simulink model "sampleModel133"  (R2021b)
settings: Solver=VariableStepAuto  StartTime=0.0  StopTime=10.0  RelTol=1e-3
libraries: simulink x4
settings Model: Creator=user  LastModifiedBy=user

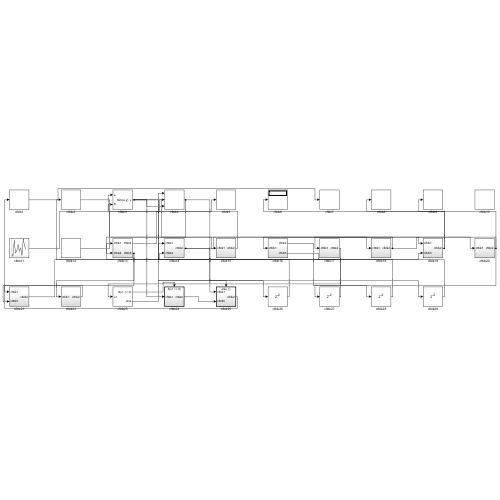
[thumbnail: Simulink's stored preview of the top-level diagram]
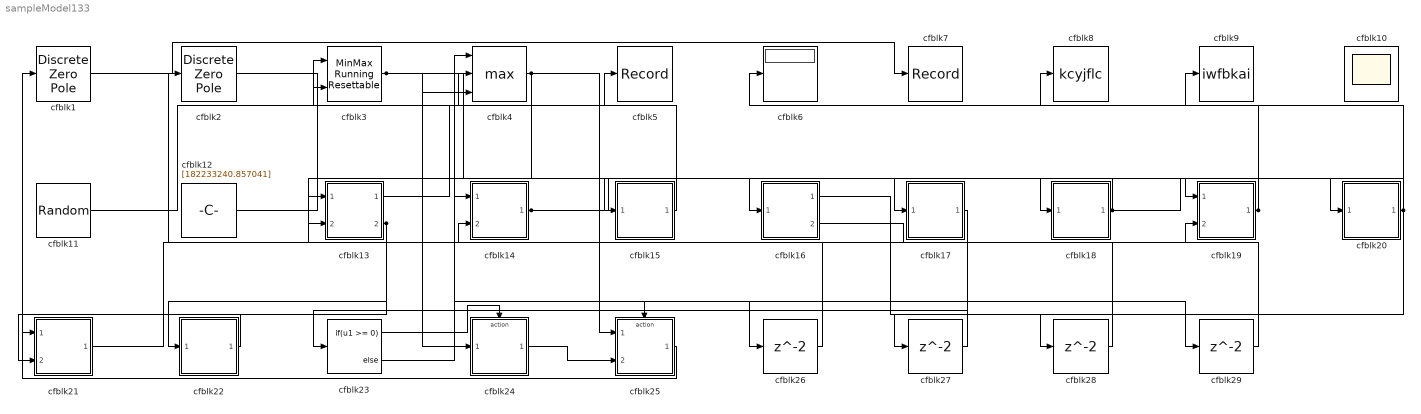
== system sampleModel133 ==
  cfblk1 : DiscreteZeroPole  Poles=[0 0.5]  Gain=1
  cfblk10 : Scope
      settings: Floating=on
  cfblk11 : UniformRandomNumber  Minimum=[-6625192953.180672]  Maximum=[659722112.246496]  Seed=[92829086.000000]  SampleTime=0.1
  cfblk12 : Constant  Value=[182233240.857041]  SampleTime=1
  cfblk13 : Subsystem
  cfblk14 : Subsystem
  cfblk15 : Subsystem
  cfblk16 : Subsystem
  cfblk17 : Subsystem
  cfblk18 : Subsystem
  cfblk19 : Subsystem
  cfblk2 : DiscreteZeroPole  Poles=[0 0.5]  Gain=1
  cfblk20 : Subsystem
  cfblk21 : Subsystem
  cfblk22 : Subsystem
  cfblk23 : If  IfExpression=u1 >= 0  SampleTime=1
  cfblk24 : Subsystem  TreatAsAtomicUnit=on
  cfblk25 : Subsystem  TreatAsAtomicUnit=on
  cfblk{26..29} (4 alike) : Delay  SampleTime=1
  cfblk3 : simulink/Math Operations/MinMax Running Resettable  Function=min  vinit=0.0
  cfblk4 : MinMax  Function=max  Inputs=3
  cfblk5 : Record  FileSettingsInternal="{\"entries\":[{\"content\":{\"excelSettings\":{\"content\":{},\"type\":\"Streamout.ExcelSettings\"}},\"type\":\"Streamout.FileSettingStorage\",\"uuid\":\"0f116b82-28e0-41c1-9d28-ccf6914d8969\"}],\"packageUris\":[\"http://schema.mathworks.com/mf0/streamout_blocks/R2020a\"],\"version\":\"1.0\"}"  SignalsInternal="{\"entries\":[{\"content\":{\"signals\":[{\"content\":{\"blockPath\":[\"sampleModel133/cfblk5\"],\"channel\":[],\"dimensions\":[1],\"domain\":\"sampleModel133/cfblk5\",\"lineColor\":\"#ff6929\",\"plots\":[1],\"port\":1,\"sid\":[\"\"],\"signalID\":4650,\"signalName\":\"cfblk13:1\"},\"type\":\"RecordBlkView.Signal\",\"uuid\":\"5c9d4d2d-3be4-4ef9-9a8e-3bb03e591d5f\"}]},\"type\":\"RecordBlkView.InputSignals\",\"uuid\":\"da5b8e4e-e8d3-4078-99a8-ef419a7cbbc8\"}],\"packageUris\":[\"http://schema.mathworks.com/mf0/streamout_blocks/R2020a\"],\"version\":\"1.0\"}"  VisualizationBindings="{\"sparklinesplugin\":{\"info\":[{\"bindingParametersList\":[],\"subplotID\":1}]}}"
  cfblk6 : Display
  cfblk7 : Record  FileSettingsInternal="{\"entries\":[{\"content\":{\"excelSettings\":{\"content\":{},\"type\":\"Streamout.ExcelSettings\"}},\"type\":\"Streamout.FileSettingStorage\",\"uuid\":\"4582ff4c-a753-4cc0-a705-87be088536e4\"}],\"packageUris\":[\"http://schema.mathworks.com/mf0/streamout_blocks/R2020a\"],\"version\":\"1.0\"}"  SignalsInternal="{\"entries\":[{\"content\":{\"signals\":[{\"content\":{\"blockPath\":[\"sampleModel133/cfblk7\"],\"channel\":[],\"dimensions\":[1],\"domain\":\"sampleModel133/cfblk7\",\"lineColor\":\"#b746ff\",\"plots\":[1],\"port\":1,\"sid\":[\"\"],\"signalID\":4654,\"signalName\":\"cfblk1\"},\"type\":\"RecordBlkView.Signal\",\"uuid\":\"e968a7e7-b7c7-42d6-b284-279b8472955c\"}]},\"type\":\"RecordBlkView.InputSignals\",\"uuid\":\"fe7274b2-3fec-4592-8935-8bf87c9eb367\"}],\"packageUris\":[\"http://schema.mathworks.com/mf0/streamout_blocks/R2020a\"],\"version\":\"1.0\"}"  VisualizationBindings="{\"sparklinesplugin\":{\"info\":[{\"bindingParametersList\":[],\"subplotID\":1}]}}"
  cfblk8 : ToWorkspace  VariableName=kcyjflc  SaveFormat=Timeseries  SampleTime=-1
  cfblk9 : ToWorkspace  VariableName=iwfbkai  SaveFormat=Timeseries  SampleTime=-1
  wires:
  cfblk20/1(cfblk2) -> cfblk9/1, cfblk16/1(cfblk1), cfblk27/1
  cfblk1/1 -> cfblk7/1
  cfblk17/1(cfblk2) -> cfblk23/1
  cfblk25/1(cfblk2) -> cfblk1/1
  cfblk14/1(cfblk2) -> cfblk18/1(cfblk1), cfblk29/1
  cfblk13/1(cfblk2) -> cfblk5/1
  cfblk18/1(cfblk2) -> cfblk17/1(cfblk1), cfblk20/1(cfblk1)
  cfblk13/2(cfblk5) -> cfblk22/1(cfblk1), cfblk21/2(cfblk3)
  cfblk2/1 -> cfblk15/1(cfblk1)
  cfblk3/1 -> cfblk25/1(cfblk1), cfblk4/3, cfblk24/1(cfblk1), cfblk26/1
  cfblk19/1(cfblk2) -> cfblk6/1, cfblk8/1
  cfblk21/1(cfblk2) -> cfblk14/2(cfblk4)
  cfblk11/1 -> cfblk3/1
  cfblk24/1(cfblk2) -> cfblk25/2(cfblk5)
  cfblk4/1 -> cfblk19/1(cfblk1), cfblk13/2(cfblk4)
  cfblk15/1(cfblk2) -> cfblk3/2
  cfblk16/2(cfblk5) -> cfblk19/2(cfblk5)
  cfblk12/1 -> cfblk4/2
  cfblk22/1(cfblk2) -> cfblk21/1(cfblk1)
  cfblk23/1 -> cfblk24/Action
  cfblk23/2 -> cfblk25/Action
  cfblk26/1 -> cfblk2/1
  cfblk27/1 -> cfblk14/1(cfblk1)
  cfblk16/1(cfblk2) -> cfblk28/1
  cfblk28/1 -> cfblk4/1
  cfblk29/1 -> cfblk13/1(cfblk1)

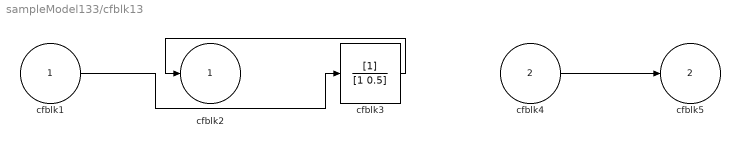
== system sampleModel133/cfblk13 ==
  cfblk1 : Inport
  cfblk4 : Inport  Port=2
  cfblk3 : DiscreteFilter  SampleTime=1
  cfblk2 : Outport
  cfblk5 : Outport  Port=2
  wires:
  cfblk3/1 -> cfblk2/1
  cfblk4/1 -> cfblk5/1
  cfblk1/1 -> cfblk3/1

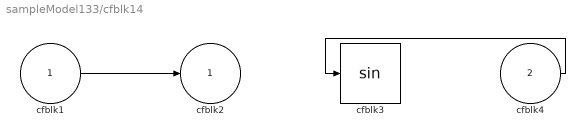
== system sampleModel133/cfblk14 ==
  cfblk1 : Inport
  cfblk4 : Inport  Port=2
  cfblk3 : Trigonometry
  cfblk2 : Outport
  wires:
  cfblk1/1 -> cfblk2/1
  cfblk4/1 -> cfblk3/1

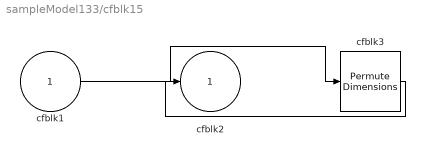
== system sampleModel133/cfblk15 ==
  cfblk1 : Inport
  cfblk3 : PermuteDimensions
  cfblk2 : Outport
  wires:
  cfblk1/1 -> cfblk3/1
  cfblk3/1 -> cfblk2/1

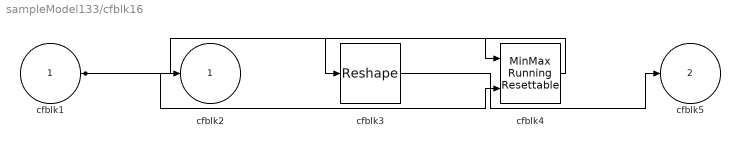
== system sampleModel133/cfblk16 ==
  cfblk1 : Inport
  cfblk3 : Reshape
  cfblk4 : simulink/Math Operations/MinMax Running Resettable  Function=min  vinit=0.0
  cfblk2 : Outport
  cfblk5 : Outport  Port=2
  wires:
  cfblk1/1 -> cfblk4/1, cfblk2/1, cfblk4/2
  cfblk3/1 -> cfblk5/1
  cfblk4/1 -> cfblk3/1

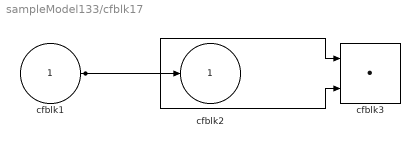
== system sampleModel133/cfblk17 ==
  cfblk1 : Inport
  cfblk3 : DotProduct  InputSameDT=on  OutDataTypeStr=Inherit: Inherit via internal rule
  cfblk2 : Outport
  wires:
  cfblk1/1 -> cfblk2/1, cfblk3/1, cfblk3/2

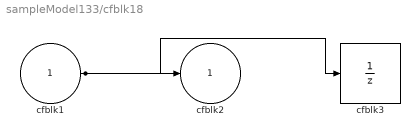
== system sampleModel133/cfblk18 ==
  cfblk1 : Inport
  cfblk3 : UnitDelay  HasFrameUpgradeWarning=on
  cfblk2 : Outport
  wires:
  cfblk1/1 -> cfblk2/1, cfblk3/1

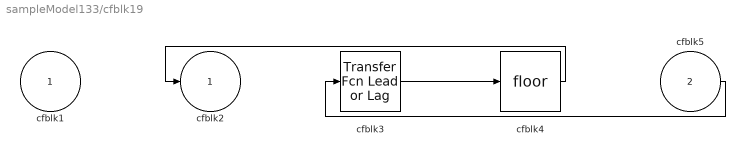
== system sampleModel133/cfblk19 ==
  cfblk1 : Inport
  cfblk5 : Inport  Port=2
  cfblk3 : simulink/Discrete/Transfer Fcn Lead or Lag  PoleZ=0.95  ZeroZ=0.75  ICPrevOutput=0.0  ICPrevInput=0.0  DoSatur=off
      settings: SourceProductBaseCode=SL
  cfblk4 : Rounding
  cfblk2 : Outport
  wires:
  cfblk3/1 -> cfblk4/1
  cfblk4/1 -> cfblk2/1
  cfblk5/1 -> cfblk3/1

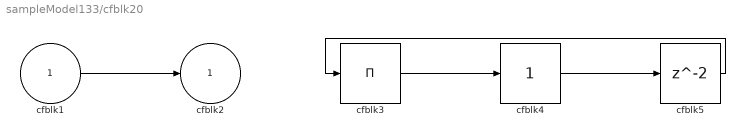
== system sampleModel133/cfblk20 ==
  cfblk1 : Inport
  cfblk3 : Product  Inputs=*
  cfblk4 : simulink/Math Operations/Slider Gain  gain=1  low=0  high=2
  cfblk5 : Delay  SampleTime=1
  cfblk2 : Outport
  wires:
  cfblk3/1 -> cfblk4/1
  cfblk1/1 -> cfblk2/1
  cfblk4/1 -> cfblk5/1
  cfblk5/1 -> cfblk3/1

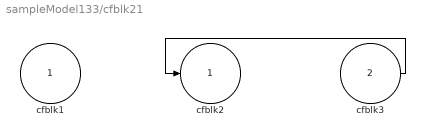
== system sampleModel133/cfblk21 ==
  cfblk1 : Inport
  cfblk3 : Inport  Port=2
  cfblk2 : Outport
  wires:
  cfblk3/1 -> cfblk2/1

== system sampleModel133/cfblk22 ==
  cfblk1 : Inport
  cfblk3 : Constant  Value=[-141337792.155833]  SampleTime=1
  cfblk2 : Outport
  wires:
  cfblk3/1 -> cfblk2/1

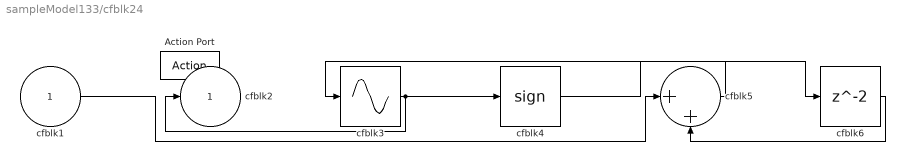
== system sampleModel133/cfblk24 ==
  cfblk1 : Inport
  Action Port : ActionPort  ActionPortLabel=if(u1 >= 0)
  cfblk3 : Sin  TimeSource=Use external signal  SampleTime=0
  cfblk4 : Signum
  cfblk5 : Sum  Inputs=|++
  cfblk6 : Delay
  cfblk2 : Outport
  wires:
  cfblk3/1 -> cfblk2/1, cfblk4/1
  cfblk1/1 -> cfblk5/1
  cfblk5/1 -> cfblk3/1
  cfblk4/1 -> cfblk6/1
  cfblk6/1 -> cfblk5/2

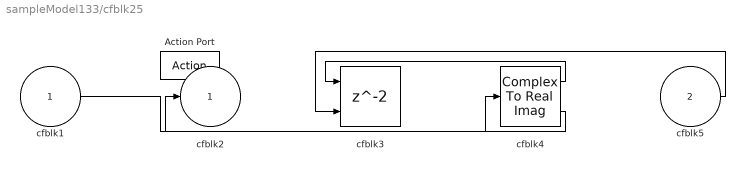
== system sampleModel133/cfblk25 ==
  cfblk1 : Inport
  cfblk5 : Inport  Port=2
  Action Port : ActionPort  ActionPortLabel=else
  cfblk3 : Delay  ShowEnablePort=on
      settings: InputPortMap=u0,e6
  cfblk4 : ComplexToRealImag
  cfblk2 : Outport
  wires:
  cfblk4/1 -> cfblk3/1
  cfblk4/2 -> cfblk2/1
  cfblk1/1 -> cfblk4/1
  cfblk5/1 -> cfblk3/2
